simulink model "Non_linear_model"  (R2020b)
settings: Solver=VariableStepAuto  StartTime=0.0  StopTime=100.0  RelTol=1e-3
values from neighbouring files (symbols this model uses):
  b1 = 5.33518    [Linearization.m]    (also in MainScript_PID.m; calib_up_up.m; tune_parameters.m = 4.8; tune_parameters_cl.m)
  b2 = 4e-05    [Linearization.m]    (also in MainScript_PID.m; calib_up_up.m; tune_parameters.m = 5e-05; tune_parameters_cl.m = 3.7644e-05)
  c1 = 0.01    [Linearization.m]    (also in MainScript_PID.m; calib_up_up.m; tune_parameters.m = -0.04; tune_parameters_cl.m = 0.025)
  c2 = 0.07    [Linearization.m]    (also in MainScript_PID.m; calib_up_up.m; tune_parameters.m = 0.0644; tune_parameters_cl.m = 0.0644)
  g = 9.81    [Linearization.m]    (also in MainScript_PID.m; calib_up_up.m; tune_parameters.m; tune_parameters_cl.m)
  I1 = 0.01076    [Linearization.m]    (also in MainScript_PID.m; calib_up_up.m; tune_parameters.m = 0.074; tune_parameters_cl.m = 0.018544)
  I2 = 0.0001    [Linearization.m]    (also in MainScript_PID.m; calib_up_up.m; tune_parameters.m; tune_parameters_cl.m = 8.3382e-05)
  km = 39.2954    [Linearization.m]    (also in MainScript_PID.m = 42.2954; calib_up_up.m; tune_parameters.m = 50; tune_parameters_cl.m)
  l1 = 0.0897    [Linearization.m]    (also in MainScript_PID.m; calib_up_up.m; tune_parameters.m = 0.1; tune_parameters_cl.m)
  m1 = 0.2    [Linearization.m]    (also in MainScript_PID.m; calib_up_up.m; tune_parameters.m = 0.125; tune_parameters_cl.m = 0.53513)
  m2 = 0.087972    [Linearization.m]    (also in MainScript_PID.m; calib_up_up.m; tune_parameters.m = 0.0528; tune_parameters_cl.m = 0.0528)
  te = 0.01    [Linearization.m]    (also in MainScript_PID.m = 0.008; calib_up_up.m; tune_parameters.m = 0.03; tune_parameters_cl.m = 0.00258)
  theta0 = [-pi;3*pi/4]    [Compute_whitebox.m]    (also in MainScript_PID.m = [-pi;     pi/4]; calib_up_up.m = [0;-pi]; tune_parameters.m = [-pi;10*pi/12]; tune_parameters_cl.m = [-pi;-pi])
  thetadot0 = [0;0]    [MainScript_PID.m]    (also in calib_up_up.m; tune_parameters.m; tune_parameters_cl.m; tune_parameters_theta1.m)
settings Model: Creator=matte  LastModifiedBy=llaporte

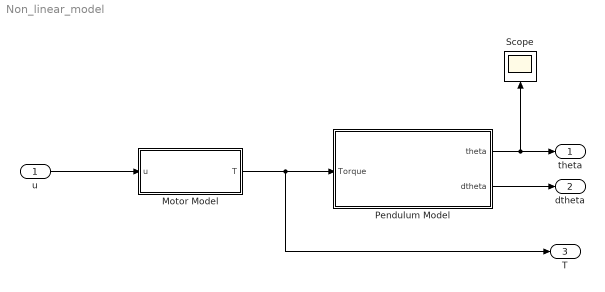
== system Non_linear_model ==
  u : Inport
  "Motor Model " : Subsystem
  Pendulum Model : Subsystem
  Scope : Scope
  theta : Outport
  dtheta : Outport  Port=2
  T : Outport  Port=3
  wires:
  Pendulum Model/1(theta) -> theta/1, Scope/1
  u/1 -> "Motor Model "/1(u)
  Pendulum Model/2(dtheta) -> dtheta/1
  "Motor Model "/1(T) -> T/1, Pendulum Model/1(Torque)

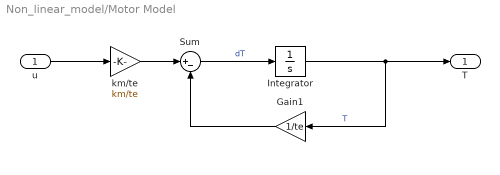
== system Non_linear_model/Motor Model  ==
  u : Inport
  Gain1 : Gain  Gain=1/te
  Integrator : Integrator
  Sum : Sum  Inputs=|+-
  "km/te " : Gain  Gain=km/te
  T : Outport
  wires:
  "km/te "/1 -> Sum/1
  u/1 -> "km/te "/1
  Integrator/1 -> T/1, Gain1/1  "T"
  Sum/1 -> Integrator/1  "dT"
  Gain1/1 -> Sum/2

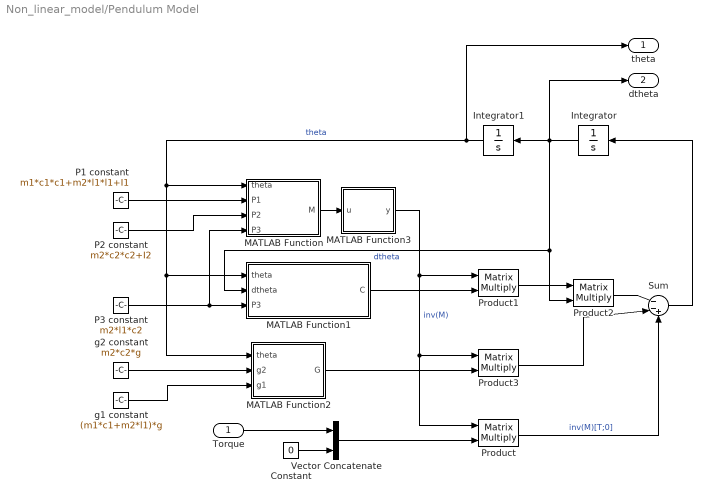
== system Non_linear_model/Pendulum Model ==
  Torque : Inport
  Constant : Constant  Value=0
  Integrator : Integrator  InitialCondition=thetadot0
  Integrator1 : Integrator  InitialCondition=theta0
  MATLAB Function : MATLAB Function  TreatAsAtomicUnit=on
  MATLAB Function1 : MATLAB Function  TreatAsAtomicUnit=on
  MATLAB Function2 : MATLAB Function  TreatAsAtomicUnit=on
  MATLAB Function3 : MATLAB Function  TreatAsAtomicUnit=on
  P1 constant : Constant  Value=m1*c1*c1+m2*l1*l1+I1
  P2 constant : Constant  Value=m2*c2*c2+I2
  P3 constant : Constant  Value=m2*l1*c2
  Product{,1..3} (4 alike) : Product  Multiplication=Matrix(*)
  Sum : Sum  Inputs=|--+
  Vector Concatenate : Concatenate
  g1 constant : Constant  Value=(m1*c1+m2*l1)*g
  g2 constant : Constant  Value=m2*c2*g
  theta : Outport
  dtheta : Outport  Port=2
  wires:
  Product/1 -> Sum/3  "inv(M)[T;0]"
  MATLAB Function3/1(y) -> Product3/1, Product/1, Product1/1  "inv(M)"
  Product1/1 -> Product2/1
  MATLAB Function/1(M) -> MATLAB Function3/1(u)
  Integrator/1 -> dtheta/1, MATLAB Function1/2(dtheta), Product2/2, Integrator1/1  "dtheta"
  Product3/1 -> Sum/2
  Integrator1/1 -> theta/1, MATLAB Function2/1(theta), MATLAB Function1/1(theta), MATLAB Function/1(theta)  "theta"
  Sum/1 -> Integrator/1
  MATLAB Function2/1(G) -> Product3/2
  MATLAB Function1/1(C) -> Product1/2
  Product2/1 -> Sum/1
  Torque/1 -> Vector Concatenate/1
  Constant/1 -> Vector Concatenate/2
  Vector Concatenate/1 -> Product/2
  g1 constant/1 -> MATLAB Function2/3(g1)
  g2 constant/1 -> MATLAB Function2/2(g2)
  P1 constant/1 -> MATLAB Function/2(P1)
  P2 constant/1 -> MATLAB Function/3(P2)
  P3 constant/1 -> MATLAB Function/4(P3), MATLAB Function1/3(P3)

== matlab function Non_linear_model/Pendulum Model/MATLAB Function ==
  data: theta input size=2; M output; P1 input; P2 input; P3 input
function M = M_matrix(theta,P1, P2, P3)
    M = [P1+P2+2*P3*cos(theta(2)) P2+P3*cos(theta(2));
         P2+P3*cos(theta(2))      P2];

== matlab function Non_linear_model/Pendulum Model/MATLAB Function1 ==
  data: theta input; C output; dtheta input; b1 parameter; b2 parameter; P3 input
function C = C_matrix(theta, dtheta,b1,b2, P3)
C = [b1-P3*dtheta(2)*sin(theta(2))  -P3*(dtheta(1)+dtheta(2))*sin(theta(2));
     P3*dtheta(1)*sin(theta(2))     b2];

== matlab function Non_linear_model/Pendulum Model/MATLAB Function2 ==
  data: theta input; G output; g2 input; g1 input
function G = G_matrix(theta,g2, g1)
G = [-g1*sin(theta(1))-g2*sin(theta(1)+theta(2));
     -g2*sin(theta(1)+theta(2))];

== matlab function Non_linear_model/Pendulum Model/MATLAB Function3 ==
  data: u input; y output
function y = inverse(u)
y = inv(u);
